simulink model "PSFB_50KHz"  (R2024a)
settings: Solver=ode23t  StartTime=0.0  StopTime=3  RelTol=1e-3
libraries: spsDiodeLib x4, spsMosfetLib x4, spsSeriesRLCBranchLib x2, spsVoltageMeasurementLib x2, spsCurrentMeasurementLib x1, spsDCVoltageSourceLib x1, spsLinearTransformerLib x1, slpidlib x1, simulink x1, spsVariableResistorLib x1, sps_lib x1
settings Model: Creator=PEG_WS1  LastModifiedBy=PEG_WS1

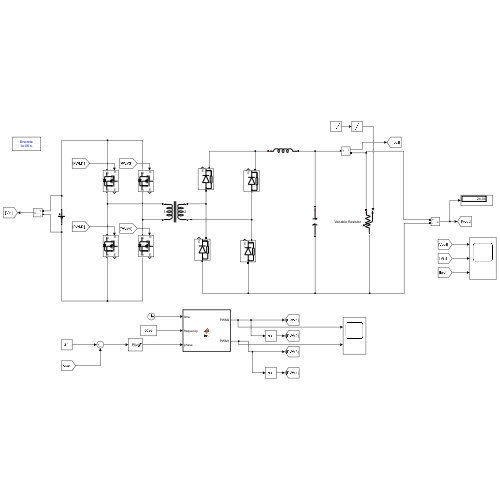
[thumbnail: Simulink's stored preview of the top-level diagram]
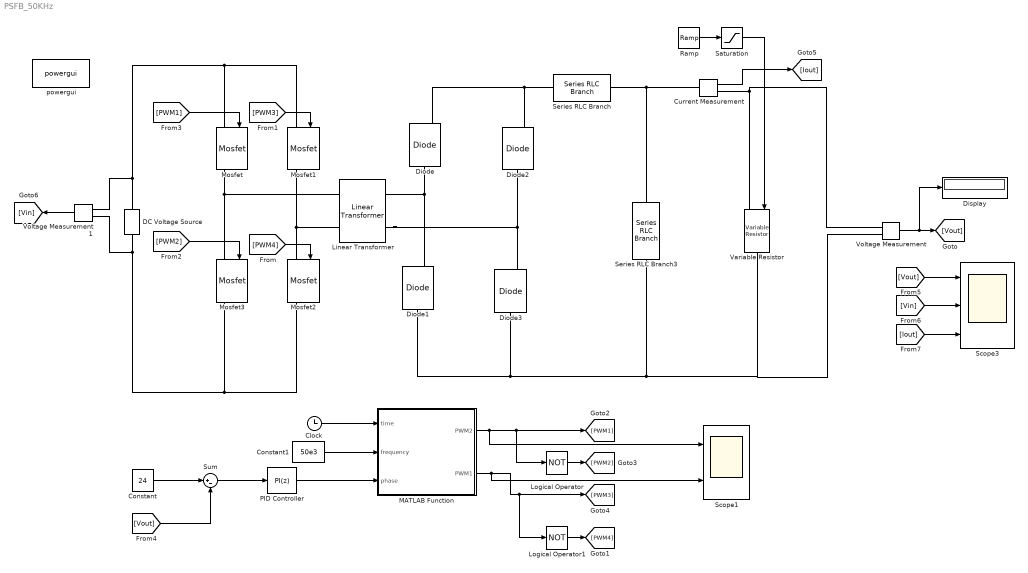
== system PSFB_50KHz ==
  Clock : Clock
  Constant : Constant  Value=24
  Constant1 : Constant  Value=50e3
  Current Measurement : spsCurrentMeasurementLib/Current Measurement  PhasorSimulation=off  OutputType=Complex  PSBequivalent=0
  DC Voltage Source : spsDCVoltageSourceLib/DC Voltage Source  Amplitude=400  Measurements=None
  Diode{,1..3} (4 alike) : spsDiodeLib/Diode  Ron=0.001  Lon=0  Vf=0.8  IC=0  UseSnubber=0  Rs=500  Cs=250e-9  Measurements=on
  Display : Display
  Linear Transformer : spsLinearTransformerLib/Linear Transformer  UNITS=SI  NominalPower=[ 1000 50e3 ]  winding1=[ 400 4.3218e-9 0.45856e-9]  winding2=[ 30 0.7938e-9 0.084225e-9]  ThreeWindings=off  winding3=[3.15e+05 0.7938 0.084225]  RmLm=[1.0804e+06 2866]  Measurements=None  DataType=on
  Logical Operator : Logic  Operator=NOT  AllPortsSameDT=off  OutDataTypeStr=boolean
  Logical Operator1 : Logic  Operator=NOT  AllPortsSameDT=off  OutDataTypeStr=boolean
  MATLAB Function : MATLAB Function  TreatAsAtomicUnit=on
  Mosfet{,1..3} (4 alike) : spsMosfetLib/Mosfet  Ron=0.1  Lon=0  Rd=0.01  Vfd=0  IC=0  Rs=1e5  Cs=inf  Measurements=on
  PID Controller : slpidlib/PID Controller  Controller=PI  Form=Parallel  TimeDomain=Discrete-time  UseExternalTs=off  SampleTime=1e-6  IntegratorMethod=Forward Euler  FilterMethod=Forward Euler  ControllerParametersSource=internal  P=7856.45  I=5645.3  UseKiTs=off  D=0  UseExternalDerivativeSource=off  N=100  UseFilter=on  TunerSelectOption=Transfer Function Based (PID Tuner App)  InitialConditionSource=internal  InitialConditionForIntegrator=0  InitialConditionForFilter=0  DifferentiatorICPrevScaledInput=0  ExternalReset=none  TrackingMode=off  Kt=1  LimitOutput=on  SatLimitsSource=internal  UpperSaturationLimit=180  LowerSaturationLimit=0  LinearizeAsGain=off  AntiWindupMode=none  Kb=1  LimitIntegrator=off  UpperIntegratorSaturationLimit=inf  LowerIntegratorSaturationLimit=-inf  POutMin=[]  POutMax=[]  IOutMin=[]  IOutMax=[]  DOutMin=[]  DOutMax=[]  NOutMin=[]  NOutMax=[]  SumOutMin=[]  SumOutMax=[]  SaturationOutMin=[]  SaturationOutMax=[]  PParamMin=[]  PParamMax=[]  IParamMin=[]  IParamMax=[]  DParamMin=[]  DParamMax=[]  NParamMin=[]  NParamMax=[]  KbParamMin=[]  KbParamMax=[]  KtParamMin=[]  KtParamMax=[]  KbOutMin=[]  KbOutMax=[]  KtOutMin=[]  KtOutMax=[]  IntegratorOutMin=[]  IntegratorOutMax=[]  FilterOutMin=[]  FilterOutMax=[]  SumI1OutMin=[]  SumI1OutMax=[]  SumI2OutMin=[]  SumI2OutMax=[]  SumI3OutMin=[]  SumI3OutMax=[]  SumI4OutMin=[]  SumI4OutMax=[]  SumDOutMin=[]  SumDOutMax=[]  DifferentiatorOutMin=[]  DifferentiatorOutMax=[]  FilterDiffOutCoefMin=[]  FilterDiffOutCoefMax=[]  ReciprocalOutMin=[]  ReciprocalOutMax=[]  SumDenOutMin=[]  SumDenOutMax=[]  SumNumOutMin=[]  SumNumOutMax=[]  DivideOutMin=[]  DivideOutMax=[]  UdiffTsProdOutMin=[]  UdiffTsProdOutMax=[]  NTsProdOutMin=[]  NTsProdOutMax=[]  UintegralTsProdOutMin=[]  UintegralTsProdOutMax=[]  UngainTsProdOutMin=[]  UngainTsProdOutMax=[]  ClampingZeroOutDataTypeStr=Inherit: Inherit via back propagation  ClampingZeroOutMin=[]  ClampingZeroOutMax=[]  FilterDenConstantOutDataTypeStr=Inherit: Inherit via back propagation  FilterDenConstantOutMin=[]  FilterDenConstantOutMax=[]  PCopyOutDataTypeStr=Inherit: Inherit via back propagation  PCopyOutMin=[]  PCopyOutMax=[]  NCopyOutDataTypeStr=Inherit: Inherit via back propagation  NCopyOutMin=[]  NCopyOutMax=[]  IntegratorContinuousStateAttributes=''  IntegratorStateMustResolveToSignalObject=off  IntegratorRTWStateStorageClass=Auto  FilterContinuousStateAttributes=''  FilterStateMustResolveToSignalObject=off  FilterRTWStateStorageClass=Auto  ParallelPVariant=InternalParameters  IdealPVariant=Disabled  IVariant=InternalParameters  DVariant=Disabled  IntegratorVariant=Discrete  SatVariant=Enabled  AWVariant=Passthrough  PCopyVariant=Disabled  TRVariant=Disabled  FdbkBlocksVariant=Forward  IdealPFdbkVariant=Disabled  SatFdbkVariant=Disabled  DerivativeFilterVariant=Disabled  NVariant=Disabled  NCopyVariant=Disabled_SignalSpec  FilterICVariant=Disabled  IntegratorICVariant=InternalICs  ExternalResetVariant=Disabled  TRSumVariant=Passthrough  SumFdbkVariant=Disabled  SumVariant=Sum_PI  TsampFilterVariant=InternalTs  TsampNgainVariant=Passthrough  TsampIntegralVariant=Disabled_SignalSpec  ExternalSaturationOutDataTypeStr=Inherit: Same as second input  DerivativeSourceVariant=Disabled
  Ramp : simulink/Sources/Ramp  slope=0.435  start=0  InitialOutput=0.86
  Saturation : Saturate  UpperLimit=1.73  LowerLimit=0.87
  Scope1 : Scope  NumInputPorts=2
  Scope3 : Scope  NumInputPorts=3
  Series RLC Branch : spsSeriesRLCBranchLib/Series RLC Branch  LConnTagsString=__new0  RConnTagsString=__new0  BranchType=L  Resistance=1  Inductance=2.7e-6  SetiL0=off  InitialCurrent=0  Capacitance=1e-6  Setx0=off  InitialVoltage=0  Measurements=None
  Series RLC Branch3 : spsSeriesRLCBranchLib/Series RLC Branch  LConnTagsString=__new0  RConnTagsString=__new0  BranchType=C  Resistance=1  Inductance=1e-3  SetiL0=off  InitialCurrent=0  Capacitance=3114.6e-6  Setx0=off  InitialVoltage=0  Measurements=None
  Sum : Sum  Inputs=|+-
  Variable Resistor : spsVariableResistorLib/Variable Resistor  Rabsmin=0.86
      settings: LibrarySourceBlock=sps_lib/Passives/Variable Resistor
  Voltage Measurement : spsVoltageMeasurementLib/Voltage Measurement  PhasorSimulation=off  OutputType=Complex  PSBequivalent=0
  Voltage Measurement1 : spsVoltageMeasurementLib/Voltage Measurement  PhasorSimulation=off  OutputType=Complex  PSBequivalent=0
  powergui : sps_lib/powergui  Priority=1  SimulationMode=Discrete  SampleTime=1e-6  frequency=60  Iterations=50  frequencyindice=0  Pbase=100e6  ErrMax=1e-4  UnitsV=kV  UnitsW=MW  buscounter=0  FunctionMessages=off  echomessages=off  EnableUseOfTLC=off  CurrentSourceSwitches=off  DisableSnubberDevices=off  DisableRonSwitches=off  DisableVfSwitches=off  DisplayEquations=off  AutomaticDiscreteSolvers=off  SolverType=Tustin/Backward Euler (TBE)  Interpol=off  ExternalGateDelay=off  methode=off  Ts=100  x0status=blocks  SPID=on  SwTol=0  HookPort=off  NonlinearTolerance=1e-4  nMaxIteration=100  ContinueOnMaxIteration=off  RestoreLinks=warning  ResistiveCurrentMeasurement=off  Frange=[0:2:500]  Ylog=off  Xlog=on  ShowGrid=off  save=off  variable=ZData  structure=0  ZoomFFT=off  StartTime=0.0  cycles=1  DisplayStyle=1  fundamental=60  FreqAxis=off  MaxFrequency=1000  frequencyindicesteady=1  RmsSteady=1  display=off
  wires:
  Voltage Measurement/1 -> Display/1, [Vout]
  Constant/1 -> Sum/1
  [Vout] -> Sum/2
  Sum/1 -> PID Controller/1
  PID Controller/1 -> MATLAB Function/3(phase)
  Constant1/1 -> MATLAB Function/2(frequency)
  Clock/1 -> MATLAB Function/1(time)
  MATLAB Function/1(PWM2) -> Scope1/1, Logical Operator/1, [PWM1]
  Logical Operator/1 -> [PWM2]
  MATLAB Function/2(PWM1) -> Scope1/2, Logical Operator1/1, [PWM3]
  Logical Operator1/1 -> [PWM4]
  [PWM1] -> Mosfet/1
  [PWM3] -> Mosfet1/1
  [PWM2] -> Mosfet3/1
  [PWM4] -> Mosfet2/1
  Ramp/1 -> Saturation/1
  Saturation/1 -> Variable Resistor/1
  Current Measurement/1 -> [Iout]
  Voltage Measurement1/1 -> [Vin]
  [Vout] -> Scope3/1
  [Vin] -> Scope3/2
  [Iout] -> Scope3/3
  connections:
  DC Voltage Source/RConn1 -- Voltage Measurement1/LConn1 -- Mosfet/LConn1 -- Mosfet1/LConn1
  Mosfet/RConn1 -- Linear Transformer/LConn1 -- Mosfet3/LConn1
  Mosfet1/RConn1 -- Linear Transformer/LConn2 -- Mosfet2/LConn1
  DC Voltage Source/LConn1 -- Voltage Measurement1/LConn2 -- Mosfet3/RConn1 -- Mosfet2/RConn1
  Diode1/RConn1 -- Linear Transformer/RConn1 -- Diode/LConn1
  Diode3/RConn1 -- Linear Transformer/RConn2 -- Diode2/LConn1
  Diode/RConn1 -- Diode2/RConn1 -- Series RLC Branch/LConn1
  Current Measurement/LConn1 -- Series RLC Branch3/LConn1 -- Series RLC Branch/RConn1
  Series RLC Branch3/RConn1 -- Diode3/LConn1 -- Diode1/LConn1 -- Variable Resistor/RConn1 -- Voltage Measurement/LConn2
  Voltage Measurement/LConn1 -- Current Measurement/RConn1 -- Variable Resistor/LConn1

== matlab function PSFB_50KHz/MATLAB Function ==
  data: time input; frequency input; phase input; PWM2 output; PWM1 output
function [PWM2, PWM1] = fcn(time,frequency,phase)
Tswitching = 1/frequency;
PWM1=0;
PWM2=0;
y1=mod(time,Tswitching);
if y1<Tswitching/2
    PWM1=1;
end
t_phi = Tswitching*phase/360;
y2=mod(time+t_phi,Tswitching);
if y2<Tswitching/2
    PWM2=1;
end
